simulink model "untitled33"  (R2020a)
settings: Solver=VariableStepAuto  StartTime=0.0  StopTime=.05  RelTol=1e-3
libraries: simulink x1, powerlib_meascontrol x1
settings Model: Creator=hp  LastModifiedBy=hp

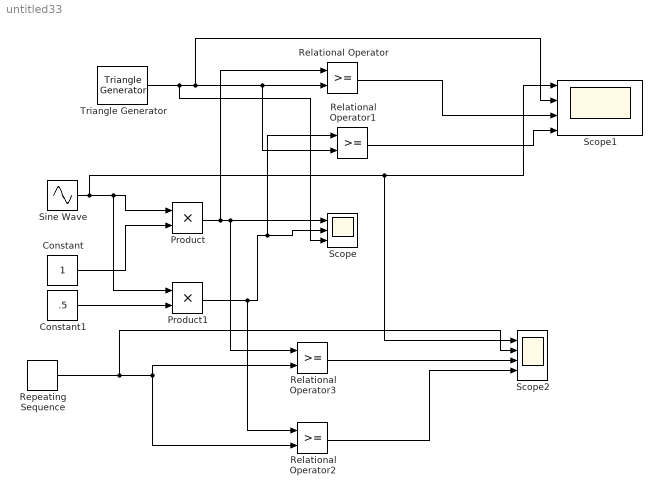
== system untitled33 ==
  Constant : Constant
  Constant1 : Constant  Value=.5
  Product : Product
  Product1 : Product
  Relational Operator{,1..3} (4 alike) : RelationalOperator  OutDataTypeStr=boolean  RndMeth=Simplest
  Repeating Sequence : simulink/Sources/Repeating Sequence  rep_seq_t=[0 .0005 .001]  rep_seq_y=[0 1 0]
  Scope : Scope  NumInputPorts=3
  Scope1 : Scope  NumInputPorts=4
  Scope2 : Scope  NumInputPorts=4
  Sine Wave : Sin  Frequency=2*pi*50  SampleTime=0
  Triangle Generator : powerlib_meascontrol/Pulse & Signal Generators/Triangle Generator  Freq=5e2  Phase=90  Ts=0
  wires:
  Product/1 -> Relational Operator/1, Relational Operator3/1, Scope/1
  Product1/1 -> Relational Operator2/1, Relational Operator1/1, Scope/2
  Sine Wave/1 -> Scope1/1, Scope2/1, Product1/1, Product/1
  Constant/1 -> Product/2
  Constant1/1 -> Product1/2
  Triangle Generator/1 -> Scope/3, Scope1/2, Relational Operator1/2, Relational Operator/2
  Relational Operator1/1 -> Scope1/4
  Repeating Sequence/1 -> Scope2/2, Relational Operator2/2, Relational Operator3/2
  Relational Operator3/1 -> Scope2/3
  Relational Operator2/1 -> Scope2/4
  Relational Operator/1 -> Scope1/3
